simulink model "V2G_System_iPI_Control_Optimized"  (R2025a)
settings: Solver=VariableStepAuto  StartTime=0.0  StopTime=1  RelTol=1e-3
undefined symbols (not defined in the file or in its folder): alpha, Ion, Ki, Kp, Lithium
libraries: spsSeriesRLCBranchLib x16, spsIGBTDiodeLib x12, spsCurrentMeasurementLib x6, slpidlib x4, spsBatteryLib x3, spsPWMGeneratorDCDCLib x3, spsAlphaBetaZerotodq0Lib x3, spsPWMGenerator2LevelLib x1, spsabctoAlphaBetaZeroLib x1, spsdq0toabcLib x1, simulink x1, spsThreePhaseVIMeasurementLib x1
settings Model: Creator=volet  LastModifiedBy=Nripace

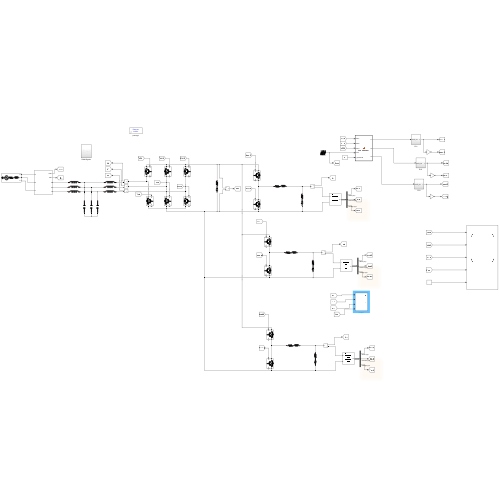
[thumbnail: Simulink's stored preview of the top-level diagram]
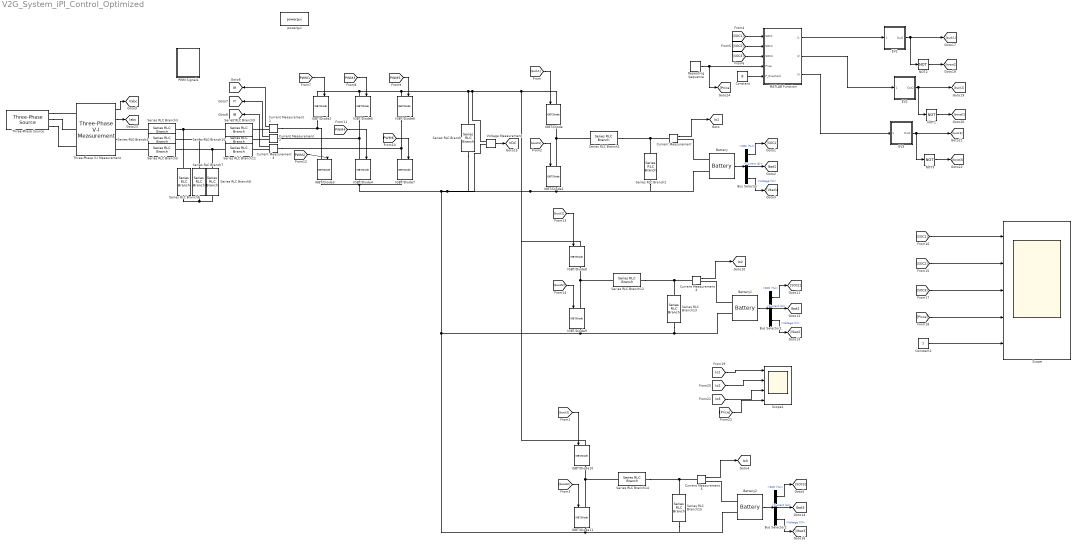
== system V2G_System_iPI_Control_Optimized ==
  Battery : spsBatteryLib/Battery  BatType=Lithium-Ion  NomV=360  NomQ=300  SOC=35  Batt_Tr=1  PresetModel=on  MaxQ=300  MinV=270  FullV=419.0354  Dis_rate=130.4348  R=0.012  Normal_OP=271.3043  expZone="[388.9389      14.73913]"
  Battery1 : spsBatteryLib/Battery  BatType=Lithium-Ion  NomV=360  NomQ=300  SOC=50  Batt_Tr=1  PresetModel=on  MaxQ=300  MinV=270  FullV=419.0354  Dis_rate=130.4348  R=0.012  Normal_OP=271.3043  expZone="[388.9389      14.73913]"
  Battery2 : spsBatteryLib/Battery  BatType=Lithium-Ion  NomV=360  NomQ=300  SOC=75  Batt_Tr=1  PresetModel=on  MaxQ=300  MinV=270  FullV=419.0354  Dis_rate=130.4348  R=0.012  Normal_OP=271.3043  expZone="[388.9389      14.73913]"
  Bus Selector : BusSelector  OutputSignals=SOC (%),Current (A),Voltage (V)
  Bus Selector1 : BusSelector  OutputSignals=SOC (%),Current (A),Voltage (V)
  Bus Selector2 : BusSelector  OutputSignals=SOC (%),Current (A),Voltage (V)
  Constant : Constant  Value=8
  Constant1 : Constant  Value=7
  Current Measurement{,1..5} (6 alike) : spsCurrentMeasurementLib/Current Measurement  PhasorSimulation=off  OutputType=Complex  PSBequivalent=0
  EV1 : Subsystem
  EV2 : Subsystem
  EV3 : Subsystem
  IGBT/Diode{,1..11} (12 alike) : spsIGBTDiodeLib/IGBT//Diode  Ron=1e-3  Rs=1e5  Cs=inf  Measurements=on
  MATLAB Function : MATLAB Function  TreatAsAtomicUnit=on
  NOT1 : Logic  Operator=NOT  IconShape=distinctive  AllPortsSameDT=off  OutDataTypeStr=boolean
  NOT2 : Logic  Operator=NOT  IconShape=distinctive  AllPortsSameDT=off  OutDataTypeStr=boolean
  NOT3 : Logic  Operator=NOT  IconShape=distinctive  AllPortsSameDT=off  OutDataTypeStr=boolean
  PWM Signals : Subsystem
  Repeating Sequence : simulink/Sources/Repeating Sequence  rep_seq_t=[0 0.1 0.2 0.3 0.4 0.5 0.6 0.7 0.8 0.9 1]  rep_seq_y=[6 3.5 8 4.3 6.7 9 8.4 8.8 11 10 9]
  Scope : Scope  NumInputPorts=5
      settings: ActiveDisplayYMinimum=17.794745633890674  ActiveDisplayYMaximum=17.796976065870169
  Scope1 : Scope  NumInputPorts=4
      settings: ActiveDisplayYMinimum=-282.20581600394803  ActiveDisplayYMaximum=129.45342106737178
  Series RLC Branch : spsSeriesRLCBranchLib/Series RLC Branch  LConnTagsString=__new0  RConnTagsString=__new0  BranchType=RC  Resistance=1e-3  Inductance=1e-3  SetiL0=off  InitialCurrent=0  Capacitance=5600e-6  Setx0=on  InitialVoltage=800  Measurements=None
  Series RLC Branch1 : spsSeriesRLCBranchLib/Series RLC Branch  LConnTagsString=__new0  RConnTagsString=__new0  BranchType=RL  Resistance=1e-4  Inductance=20e-3  SetiL0=off  InitialCurrent=0  Capacitance=1000e-6  Setx0=off  InitialVoltage=0  Measurements=None
  Series RLC Branch{3..5,9..11} (6 alike) : spsSeriesRLCBranchLib/Series RLC Branch  LConnTagsString=__new0  RConnTagsString=__new0  BranchType=L  Resistance=1  Inductance=5e-3  SetiL0=off  InitialCurrent=0  Capacitance=1e-6  Setx0=off  InitialVoltage=0  Measurements=None
  Series RLC Branch12 : spsSeriesRLCBranchLib/Series RLC Branch  LConnTagsString=__new0  RConnTagsString=__new0  BranchType=RL  Resistance=1e-4  Inductance=20e-3  SetiL0=off  InitialCurrent=0  Capacitance=1000e-6  Setx0=off  InitialVoltage=0  Measurements=None
  Series RLC Branch13 : spsSeriesRLCBranchLib/Series RLC Branch  LConnTagsString=__new0  RConnTagsString=__new0  BranchType=RC  Resistance=1e-4  Inductance=1e-3  SetiL0=off  InitialCurrent=0  Capacitance=0.625e-6  Setx0=off  InitialVoltage=0  Measurements=None
  Series RLC Branch14 : spsSeriesRLCBranchLib/Series RLC Branch  LConnTagsString=__new0  RConnTagsString=__new0  BranchType=RL  Resistance=1e-4  Inductance=20e-3  SetiL0=off  InitialCurrent=0  Capacitance=1000e-6  Setx0=off  InitialVoltage=0  Measurements=None
  Series RLC Branch15 : spsSeriesRLCBranchLib/Series RLC Branch  LConnTagsString=__new0  RConnTagsString=__new0  BranchType=RC  Resistance=1e-4  Inductance=1e-3  SetiL0=off  InitialCurrent=0  Capacitance=0.625e-6  Setx0=off  InitialVoltage=0  Measurements=None
  Series RLC Branch2 : spsSeriesRLCBranchLib/Series RLC Branch  LConnTagsString=__new0  RConnTagsString=__new0  BranchType=RC  Resistance=1e-4  Inductance=1e-3  SetiL0=off  InitialCurrent=0  Capacitance=0.625e-6  Setx0=off  InitialVoltage=0  Measurements=None
  Series RLC Branch6 : spsSeriesRLCBranchLib/Series RLC Branch  LConnTagsString=__new0  RConnTagsString=__new0  BranchType=C  Resistance=1  Inductance=5e-3  SetiL0=off  InitialCurrent=0  Capacitance=30e-6  Setx0=off  InitialVoltage=0  Measurements=None
  Series RLC Branch7 : spsSeriesRLCBranchLib/Series RLC Branch  LConnTagsString=__new0  RConnTagsString=__new0  BranchType=C  Resistance=1  Inductance=5e-3  SetiL0=off  InitialCurrent=0  Capacitance=30e-6  Setx0=off  InitialVoltage=0  Measurements=None
  Series RLC Branch8 : spsSeriesRLCBranchLib/Series RLC Branch  LConnTagsString=__new0  RConnTagsString=__new0  BranchType=C  Resistance=1  Inductance=5e-3  SetiL0=off  InitialCurrent=0  Capacitance=30e-6  Setx0=off  InitialVoltage=0  Measurements=None
  Three-Phase V-I Measurement : spsThreePhaseVIMeasurementLib/Three-Phase V-I Measurement  VoltageMeasurement=phase-to-ground  SetLabelV=off  LabelV=Vabc  Vpu=off  VpuLL=off  CurrentMeasurement=yes  SetLabelI=off  LabelI=Iabc  Ipu=off  Pbase=100e6  Vbase=500e3  OutputType=Complex  PhasorSimulation=off  PSBequivalent=0
  Three-Phase Source : spsThreePhaseSourceLib/Three-Phase Source  InternalConnection=Yg  VoltagePhases=off  Voltage=415  PhaseAngle=0  Voltage_phases=[25e3 25e3 25e3]/sqrt(3)  PhaseAngles_phases=[0 -120 +120]  Frequency=50  NonIdealSource=on  SpecifyImpedance=off  Resistance=0.8929e-3  Inductance=16.58e-9  ShortCircuitLevel=100e6  BaseVoltage=415  XRratio=7  BusType=swing  Pref=10e3  Qref=0  Prefabc=[10e3, 10e3, 10e3]  Qrefabc=[0, 0, 0]  Qmin=-inf  Qmax=inf
  Voltage Measurement : spsVoltageMeasurementLib/Voltage Measurement  PhasorSimulation=off  OutputType=Complex  PSBequivalent=0
  powergui : sps_lib/powergui  Priority=1  SimulationMode=Discrete  SampleTime=1e-6  frequency=60  Iterations=50  frequencyindice=0  Pbase=100e6  ErrMax=1e-4  UnitsV=kV  UnitsW=MW  buscounter=0  FunctionMessages=off  echomessages=off  EnableUseOfTLC=off  CurrentSourceSwitches=off  DisableSnubberDevices=off  DisableRonSwitches=off  DisableVfSwitches=off  DisplayEquations=off  AutomaticDiscreteSolvers=off  SolverType=Tustin/Backward Euler (TBE)  Interpol=off  ExternalGateDelay=off  methode=off  Ts=100  x0status=blocks  SPID=on  SwTol=0  HookPort=off  NonlinearTolerance=1e-4  nMaxIteration=100  ContinueOnMaxIteration=off  RestoreLinks=warning  ResistiveCurrentMeasurement=off  Frange=[0:2:500]  Ylog=off  Xlog=on  ShowGrid=off  save=off  variable=ZData  structure=0  ZoomFFT=off  StartTime=0.0  cycles=1  DisplayStyle=1  fundamental=60  FreqAxis=off  MaxFrequency=1000  frequencyindicesteady=1  RmsSteady=1  display=off
  tag scope: IB=global, IR=global, IY=global, Iabc=global, Ibat1=global, Ibat2=global, Ibat3=global, Io1=global, Io2=global, Io3=global, VDC=global, Vabc=global
  wires:
  [boost3] -> IGBT/Diode11/1
  [Io3] -> Scope1/3
  Voltage Measurement/1 -> [VDC]
  [PWM3] -> IGBT/Diode5/1
  Bus Selector2/1 -> [SOC3]  "<SOC (%)>"
  Bus Selector2/3 -> [Vbat3]  "<Voltage (V)>"
  [PWM5] -> IGBT/Diode6/1
  [PWM4] -> IGBT/Diode4/1
  [SOC3] -> Scope/3
  MATLAB Function/3(I3) -> EV3/1(Price_ref)
  Three-Phase V-I Measurement/1 -> [Vabc]
  Bus Selector2/2 -> [Ibat3]  "<Current (A)>"
  Current Measurement1/1 -> [IR]
  [Io1] -> Scope1/1
  Bus Selector1/3 -> [Vbat2]  "<Voltage (V)>"
  [SOC3] -> MATLAB Function/3(SOC3)
  Current Measurement4/1 -> [Io2]
  Bus Selector/3 -> [Vbat1]  "<Voltage (V)>"
  EV1/1(Out2) -> [buck1], NOT2/1
  [boost2] -> IGBT/Diode9/1
  MATLAB Function/2(I2) -> EV2/1(Price_ref)
  NOT1/1 -> [boost2]
  [SOC2] -> Scope/2
  [boost1] -> IGBT/Diode1/1
  EV3/1(Out2) -> [buck3], NOT3/1
  Bus Selector/2 -> [Ibat1]  "<Current (A)>"
  [PWM6] -> IGBT/Diode7/1
  Repeating Sequence/1 -> MATLAB Function/4(Price), [Price]
  Three-Phase V-I Measurement/2 -> [Iabc]
  [SOC1] -> MATLAB Function/1(SOC1)
  Constant/1 -> MATLAB Function/5(P_threshold)
  NOT3/1 -> [boost3]
  Bus Selector/1 -> [SOC1]  "<SOC (%)>"
  NOT2/1 -> [boost1]
  [buck2] -> IGBT/Diode8/1
  [Price] -> Scope/4
  Bus Selector1/1 -> [SOC2]  "<SOC (%)>"
  [SOC1] -> Scope/1
  Current Measurement3/1 -> [IB]
  [buck3] -> IGBT/Diode10/1
  MATLAB Function/1(I1) -> EV1/1(Price_ref)
  Current Measurement2/1 -> [IY]
  Battery2/1 -> Bus Selector2/1
  Current Measurement/1 -> [Io1]
  [PWM2] -> IGBT/Diode3/1
  Battery/1 -> Bus Selector/1
  Current Measurement5/1 -> [Io3]
  [Io2] -> Scope1/2
  Bus Selector1/2 -> [Ibat2]  "<Current (A)>"
  [SOC2] -> MATLAB Function/2(SOC2)
  [PWM1] -> IGBT/Diode2/1
  EV2/1(Out2) -> [buck2], NOT1/1
  Battery1/1 -> Bus Selector1/1
  [buck1] -> IGBT/Diode/1
  Constant1/1 -> Scope/5
  [Price] -> Scope1/4
  connections:
  Series RLC Branch14/RConn1 -- Current Measurement5/LConn1 -- Series RLC Branch15/LConn1
  Series RLC Branch13/RConn1 -- Battery1/LConn2 -- IGBT/Diode9/RConn1 -- IGBT/Diode11/RConn1 -- Battery2/LConn2 -- Series RLC Branch15/RConn1 -- IGBT/Diode3/RConn1 -- IGBT/Diode4/RConn1 -- IGBT/Diode7/RConn1 -- Series RLC Branch/RConn1 -- Voltage Measurement/LConn2 -- Battery/LConn2 -- Series RLC Branch2/RConn1 -- IGBT/Diode1/RConn1
  IGBT/Diode5/LConn1 -- IGBT/Diode10/LConn1 -- IGBT/Diode8/LConn1 -- IGBT/Diode/LConn1 -- Voltage Measurement/LConn1 -- Series RLC Branch/LConn1 -- IGBT/Diode6/LConn1 -- IGBT/Diode2/LConn1
  IGBT/Diode9/LConn1 -- Series RLC Branch12/LConn1 -- IGBT/Diode8/RConn1
  IGBT/Diode11/LConn1 -- Series RLC Branch14/LConn1 -- IGBT/Diode10/RConn1
  Series RLC Branch6/RConn1 -- Series RLC Branch7/RConn1 -- Series RLC Branch8/RConn1
  IGBT/Diode1/LConn1 -- Series RLC Branch1/LConn1 -- IGBT/Diode/RConn1
  IGBT/Diode5/RConn1 -- Current Measurement2/LConn1 -- IGBT/Diode4/LConn1
  Series RLC Branch3/RConn1 -- Series RLC Branch6/LConn1 -- Series RLC Branch9/LConn1
  IGBT/Diode2/RConn1 -- Current Measurement1/LConn1 -- IGBT/Diode3/LConn1
  Series RLC Branch7/LConn1 -- Series RLC Branch4/RConn1 -- Series RLC Branch10/LConn1
  IGBT/Diode6/RConn1 -- Current Measurement3/LConn1 -- IGBT/Diode7/LConn1
  Series RLC Branch8/LConn1 -- Series RLC Branch5/RConn1 -- Series RLC Branch11/LConn1
  Series RLC Branch1/RConn1 -- Current Measurement/LConn1 -- Series RLC Branch2/LConn1
  Series RLC Branch12/RConn1 -- Current Measurement4/LConn1 -- Series RLC Branch13/LConn1
  Current Measurement3/RConn1 -- Series RLC Branch11/RConn1
  Battery/LConn1 -- Current Measurement/RConn1
  Three-Phase Source/RConn3 -- Three-Phase V-I Measurement/LConn3
  Current Measurement2/RConn1 -- Series RLC Branch10/RConn1
  Three-Phase Source/RConn2 -- Three-Phase V-I Measurement/LConn2
  Series RLC Branch3/LConn1 -- Three-Phase V-I Measurement/RConn1
  Series RLC Branch4/LConn1 -- Three-Phase V-I Measurement/RConn2
  Three-Phase Source/RConn1 -- Three-Phase V-I Measurement/LConn1
  Battery2/LConn1 -- Current Measurement5/RConn1
  Current Measurement1/RConn1 -- Series RLC Branch9/RConn1
  Battery1/LConn1 -- Current Measurement4/RConn1
  Series RLC Branch5/LConn1 -- Three-Phase V-I Measurement/RConn3

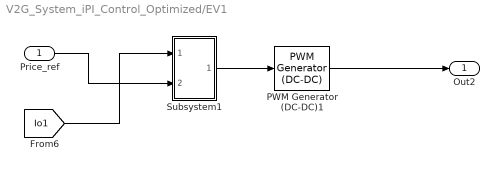
== system V2G_System_iPI_Control_Optimized/EV1 ==
  Price_ref : Inport
  PWM Generator (DC-DC)1 : spsPWMGeneratorDCDCLib/PWM Generator (DC-DC)  Fsw=10000  Ts=0
  Subsystem1 : Subsystem
  Out2 : Outport  VectorParamsAs1DForOutWhenUnconnected=off
  wires:
  Subsystem1/1(Out1) -> PWM Generator (DC-DC)1/1
  PWM Generator (DC-DC)1/1 -> Out2/1
  [Io1] -> Subsystem1/1(Price_ref)
  Price_ref/1 -> Subsystem1/2(In2)

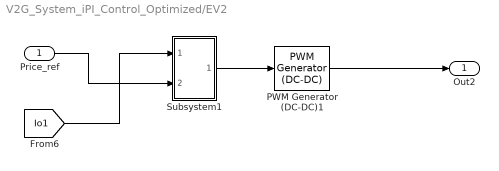
== system V2G_System_iPI_Control_Optimized/EV2 ==
  Price_ref : Inport
  PWM Generator (DC-DC)1 : spsPWMGeneratorDCDCLib/PWM Generator (DC-DC)  Fsw=10000  Ts=0
  Subsystem1 : Subsystem
  Out2 : Outport  VectorParamsAs1DForOutWhenUnconnected=off
  wires:
  Subsystem1/1(Out1) -> PWM Generator (DC-DC)1/1
  PWM Generator (DC-DC)1/1 -> Out2/1
  [Io1] -> Subsystem1/1(Price_ref)
  Price_ref/1 -> Subsystem1/2(In2)

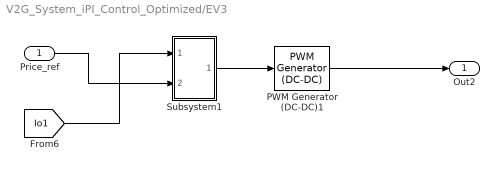
== system V2G_System_iPI_Control_Optimized/EV3 ==
  Price_ref : Inport
  PWM Generator (DC-DC)1 : spsPWMGeneratorDCDCLib/PWM Generator (DC-DC)  Fsw=10000  Ts=0
  Subsystem1 : Subsystem
  Out2 : Outport  VectorParamsAs1DForOutWhenUnconnected=off
  wires:
  Price_ref/1 -> Subsystem1/2(In2)
  [Io1] -> Subsystem1/1(Price_ref)
  PWM Generator (DC-DC)1/1 -> Out2/1
  Subsystem1/1(Out1) -> PWM Generator (DC-DC)1/1

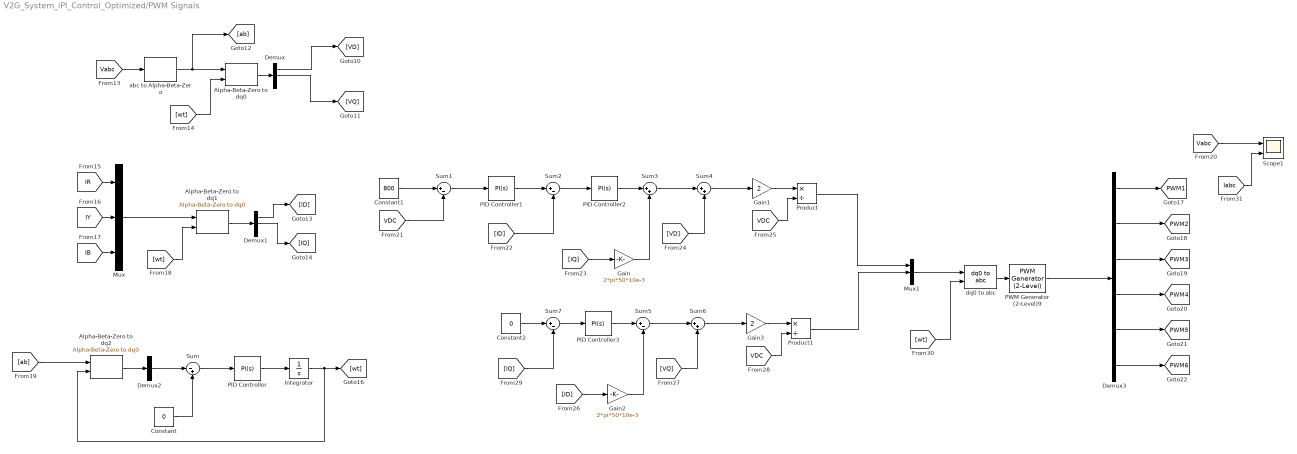
== system V2G_System_iPI_Control_Optimized/PWM Signals ==
  Alpha-Beta-Zero to dq0 : spsAlphaBetaZerotodq0Lib/Alpha-Beta-Zero to dq0  Alignment=90 degrees behind phase A axis
  Alpha-Beta-Zero to dq1 : spsAlphaBetaZerotodq0Lib/Alpha-Beta-Zero to dq0  Alignment=90 degrees behind phase A axis
  Alpha-Beta-Zero to dq2 : spsAlphaBetaZerotodq0Lib/Alpha-Beta-Zero to dq0  Alignment=90 degrees behind phase A axis
  Constant : Constant  Value=0
  Constant1 : Constant  Value=800
  Constant2 : Constant  Value=0
  Demux : Demux  Outputs=3
  Demux1 : Demux  Outputs=3
  Demux2 : Demux  Outputs=3
  Demux3 : Demux  Outputs=6
  Gain : Gain  Gain=2*pi*50*10e-3
  Gain1 : Gain  Gain=2
  Gain2 : Gain  Gain=2*pi*50*10e-3
  Gain3 : Gain  Gain=2
  Integrator : Integrator
  Mux : Mux  Inputs=3
  Mux1 : Mux  Inputs=3
  PID Controller : slpidlib/PID Controller  Controller=PI  Form=Parallel  TimeDomain=Continuous-time  UseExternalTs=off  SampleTime=-1  IntegratorMethod=Forward Euler  FilterMethod=Forward Euler  ControllerParametersSource=internal  P=10  I=50000  UseKiTs=off  D=0  UseExternalDerivativeSource=off  N=100  UseFilter=on  TunerSelectOption=Transfer Function Based (PID Tuner App)  InitialConditionSource=internal  InitialConditionForIntegrator=0  InitialConditionForFilter=0  DifferentiatorICPrevScaledInput=0  ExternalReset=none  TrackingMode=off  Kt=1  LimitOutput=off  SatLimitsSource=internal  UpperSaturationLimit=inf  LowerSaturationLimit=-inf  LinearizeAsGain=on  AntiWindupMode=none  Kb=1  LimitIntegrator=off  UpperIntegratorSaturationLimit=inf  LowerIntegratorSaturationLimit=-inf  POutMin=[]  POutMax=[]  IOutMin=[]  IOutMax=[]  DOutMin=[]  DOutMax=[]  NOutMin=[]  NOutMax=[]  SumOutMin=[]  SumOutMax=[]  SaturationOutMin=[]  SaturationOutMax=[]  PParamMin=[]  PParamMax=[]  IParamMin=[]  IParamMax=[]  DParamMin=[]  DParamMax=[]  NParamMin=[]  NParamMax=[]  KbParamMin=[]  KbParamMax=[]  KtParamMin=[]  KtParamMax=[]  KbOutMin=[]  KbOutMax=[]  KtOutMin=[]  KtOutMax=[]  IntegratorOutMin=[]  IntegratorOutMax=[]  FilterOutMin=[]  FilterOutMax=[]  SumI1OutMin=[]  SumI1OutMax=[]  SumI2OutMin=[]  SumI2OutMax=[]  SumI3OutMin=[]  SumI3OutMax=[]  SumI4OutMin=[]  SumI4OutMax=[]  SumDOutMin=[]  SumDOutMax=[]  DifferentiatorOutMin=[]  DifferentiatorOutMax=[]  FilterDiffOutCoefMin=[]  FilterDiffOutCoefMax=[]  ReciprocalOutMin=[]  ReciprocalOutMax=[]  SumDenOutMin=[]  SumDenOutMax=[]  SumNumOutMin=[]  SumNumOutMax=[]  DivideOutMin=[]  DivideOutMax=[]  UdiffTsProdOutMin=[]  UdiffTsProdOutMax=[]  NTsProdOutMin=[]  NTsProdOutMax=[]  UintegralTsProdOutMin=[]  UintegralTsProdOutMax=[]  UngainTsProdOutMin=[]  UngainTsProdOutMax=[]  ClampingZeroOutDataTypeStr=Inherit: Inherit via back propagation  ClampingZeroOutMin=[]  ClampingZeroOutMax=[]  FilterDenConstantOutDataTypeStr=Inherit: Inherit via back propagation  FilterDenConstantOutMin=[]  FilterDenConstantOutMax=[]  PCopyOutDataTypeStr=Inherit: Inherit via back propagation  PCopyOutMin=[]  PCopyOutMax=[]  NCopyOutDataTypeStr=Inherit: Inherit via back propagation  NCopyOutMin=[]  NCopyOutMax=[]  IntegratorContinuousStateAttributes=''  IntegratorStateMustResolveToSignalObject=off  IntegratorRTWStateStorageClass=Auto  FilterContinuousStateAttributes=''  FilterStateMustResolveToSignalObject=off  FilterRTWStateStorageClass=Auto  ParallelPVariant=InternalParameters  IdealPVariant=Disabled  IVariant=InternalParameters  DVariant=Disabled  IntegratorVariant=Continuous  SatVariant=Disabled  AWVariant=Passthrough  PCopyVariant=Disabled  TRVariant=Disabled  FdbkBlocksVariant=Forward  IdealPFdbkVariant=Disabled  SatFdbkVariant=Disabled  DerivativeFilterVariant=Disabled  NVariant=Disabled  NCopyVariant=Disabled_SignalSpec  FilterICVariant=Disabled  IntegratorICVariant=InternalICs  ExternalResetVariant=Disabled  TRSumVariant=Passthrough  SumFdbkVariant=Disabled  SumVariant=Sum_PI  TsampFilterVariant=InternalTs  TsampNgainVariant=Passthrough  TsampIntegralVariant=Disabled_SignalSpec  ExternalSaturationOutDataTypeStr=Inherit: Same as second input  DerivativeSourceVariant=Disabled  PreIntVariant=InternalPreInt
  PID Controller1 : slpidlib/PID Controller  Controller=PI  Form=Parallel  TimeDomain=Continuous-time  UseExternalTs=off  SampleTime=-1  IntegratorMethod=Forward Euler  FilterMethod=Forward Euler  ControllerParametersSource=internal  P=0.5  I=5  UseKiTs=off  D=0  UseExternalDerivativeSource=off  N=100  UseFilter=on  TunerSelectOption=Transfer Function Based (PID Tuner App)  InitialConditionSource=internal  InitialConditionForIntegrator=0  InitialConditionForFilter=0  DifferentiatorICPrevScaledInput=0  ExternalReset=none  TrackingMode=off  Kt=1  LimitOutput=off  SatLimitsSource=internal  UpperSaturationLimit=inf  LowerSaturationLimit=-inf  LinearizeAsGain=on  AntiWindupMode=none  Kb=1  LimitIntegrator=off  UpperIntegratorSaturationLimit=inf  LowerIntegratorSaturationLimit=-inf  POutMin=[]  POutMax=[]  IOutMin=[]  IOutMax=[]  DOutMin=[]  DOutMax=[]  NOutMin=[]  NOutMax=[]  SumOutMin=[]  SumOutMax=[]  SaturationOutMin=[]  SaturationOutMax=[]  PParamMin=[]  PParamMax=[]  IParamMin=[]  IParamMax=[]  DParamMin=[]  DParamMax=[]  NParamMin=[]  NParamMax=[]  KbParamMin=[]  KbParamMax=[]  KtParamMin=[]  KtParamMax=[]  KbOutMin=[]  KbOutMax=[]  KtOutMin=[]  KtOutMax=[]  IntegratorOutMin=[]  IntegratorOutMax=[]  FilterOutMin=[]  FilterOutMax=[]  SumI1OutMin=[]  SumI1OutMax=[]  SumI2OutMin=[]  SumI2OutMax=[]  SumI3OutMin=[]  SumI3OutMax=[]  SumI4OutMin=[]  SumI4OutMax=[]  SumDOutMin=[]  SumDOutMax=[]  DifferentiatorOutMin=[]  DifferentiatorOutMax=[]  FilterDiffOutCoefMin=[]  FilterDiffOutCoefMax=[]  ReciprocalOutMin=[]  ReciprocalOutMax=[]  SumDenOutMin=[]  SumDenOutMax=[]  SumNumOutMin=[]  SumNumOutMax=[]  DivideOutMin=[]  DivideOutMax=[]  UdiffTsProdOutMin=[]  UdiffTsProdOutMax=[]  NTsProdOutMin=[]  NTsProdOutMax=[]  UintegralTsProdOutMin=[]  UintegralTsProdOutMax=[]  UngainTsProdOutMin=[]  UngainTsProdOutMax=[]  ClampingZeroOutDataTypeStr=Inherit: Inherit via back propagation  ClampingZeroOutMin=[]  ClampingZeroOutMax=[]  FilterDenConstantOutDataTypeStr=Inherit: Inherit via back propagation  FilterDenConstantOutMin=[]  FilterDenConstantOutMax=[]  PCopyOutDataTypeStr=Inherit: Inherit via back propagation  PCopyOutMin=[]  PCopyOutMax=[]  NCopyOutDataTypeStr=Inherit: Inherit via back propagation  NCopyOutMin=[]  NCopyOutMax=[]  IntegratorContinuousStateAttributes=''  IntegratorStateMustResolveToSignalObject=off  IntegratorRTWStateStorageClass=Auto  FilterContinuousStateAttributes=''  FilterStateMustResolveToSignalObject=off  FilterRTWStateStorageClass=Auto  ParallelPVariant=InternalParameters  IdealPVariant=Disabled  IVariant=InternalParameters  DVariant=Disabled  IntegratorVariant=Continuous  SatVariant=Disabled  AWVariant=Passthrough  PCopyVariant=Disabled  TRVariant=Disabled  FdbkBlocksVariant=Forward  IdealPFdbkVariant=Disabled  SatFdbkVariant=Disabled  DerivativeFilterVariant=Disabled  NVariant=Disabled  NCopyVariant=Disabled_SignalSpec  FilterICVariant=Disabled  IntegratorICVariant=InternalICs  ExternalResetVariant=Disabled  TRSumVariant=Passthrough  SumFdbkVariant=Disabled  SumVariant=Sum_PI  TsampFilterVariant=InternalTs  TsampNgainVariant=Passthrough  TsampIntegralVariant=Disabled_SignalSpec  ExternalSaturationOutDataTypeStr=Inherit: Same as second input  DerivativeSourceVariant=Disabled  PreIntVariant=InternalPreInt
  PID Controller2 : slpidlib/PID Controller  Controller=PI  Form=Parallel  TimeDomain=Continuous-time  UseExternalTs=off  SampleTime=-1  IntegratorMethod=Forward Euler  FilterMethod=Forward Euler  ControllerParametersSource=internal  P=25  I=500  UseKiTs=off  D=0  UseExternalDerivativeSource=off  N=100  UseFilter=on  TunerSelectOption=Transfer Function Based (PID Tuner App)  InitialConditionSource=internal  InitialConditionForIntegrator=0  InitialConditionForFilter=0  DifferentiatorICPrevScaledInput=0  ExternalReset=none  TrackingMode=off  Kt=1  LimitOutput=off  SatLimitsSource=internal  UpperSaturationLimit=inf  LowerSaturationLimit=-inf  LinearizeAsGain=on  AntiWindupMode=none  Kb=1  LimitIntegrator=off  UpperIntegratorSaturationLimit=inf  LowerIntegratorSaturationLimit=-inf  POutMin=[]  POutMax=[]  IOutMin=[]  IOutMax=[]  DOutMin=[]  DOutMax=[]  NOutMin=[]  NOutMax=[]  SumOutMin=[]  SumOutMax=[]  SaturationOutMin=[]  SaturationOutMax=[]  PParamMin=[]  PParamMax=[]  IParamMin=[]  IParamMax=[]  DParamMin=[]  DParamMax=[]  NParamMin=[]  NParamMax=[]  KbParamMin=[]  KbParamMax=[]  KtParamMin=[]  KtParamMax=[]  KbOutMin=[]  KbOutMax=[]  KtOutMin=[]  KtOutMax=[]  IntegratorOutMin=[]  IntegratorOutMax=[]  FilterOutMin=[]  FilterOutMax=[]  SumI1OutMin=[]  SumI1OutMax=[]  SumI2OutMin=[]  SumI2OutMax=[]  SumI3OutMin=[]  SumI3OutMax=[]  SumI4OutMin=[]  SumI4OutMax=[]  SumDOutMin=[]  SumDOutMax=[]  DifferentiatorOutMin=[]  DifferentiatorOutMax=[]  FilterDiffOutCoefMin=[]  FilterDiffOutCoefMax=[]  ReciprocalOutMin=[]  ReciprocalOutMax=[]  SumDenOutMin=[]  SumDenOutMax=[]  SumNumOutMin=[]  SumNumOutMax=[]  DivideOutMin=[]  DivideOutMax=[]  UdiffTsProdOutMin=[]  UdiffTsProdOutMax=[]  NTsProdOutMin=[]  NTsProdOutMax=[]  UintegralTsProdOutMin=[]  UintegralTsProdOutMax=[]  UngainTsProdOutMin=[]  UngainTsProdOutMax=[]  ClampingZeroOutDataTypeStr=Inherit: Inherit via back propagation  ClampingZeroOutMin=[]  ClampingZeroOutMax=[]  FilterDenConstantOutDataTypeStr=Inherit: Inherit via back propagation  FilterDenConstantOutMin=[]  FilterDenConstantOutMax=[]  PCopyOutDataTypeStr=Inherit: Inherit via back propagation  PCopyOutMin=[]  PCopyOutMax=[]  NCopyOutDataTypeStr=Inherit: Inherit via back propagation  NCopyOutMin=[]  NCopyOutMax=[]  IntegratorContinuousStateAttributes=''  IntegratorStateMustResolveToSignalObject=off  IntegratorRTWStateStorageClass=Auto  FilterContinuousStateAttributes=''  FilterStateMustResolveToSignalObject=off  FilterRTWStateStorageClass=Auto  ParallelPVariant=InternalParameters  IdealPVariant=Disabled  IVariant=InternalParameters  DVariant=Disabled  IntegratorVariant=Continuous  SatVariant=Disabled  AWVariant=Passthrough  PCopyVariant=Disabled  TRVariant=Disabled  FdbkBlocksVariant=Forward  IdealPFdbkVariant=Disabled  SatFdbkVariant=Disabled  DerivativeFilterVariant=Disabled  NVariant=Disabled  NCopyVariant=Disabled_SignalSpec  FilterICVariant=Disabled  IntegratorICVariant=InternalICs  ExternalResetVariant=Disabled  TRSumVariant=Passthrough  SumFdbkVariant=Disabled  SumVariant=Sum_PI  TsampFilterVariant=InternalTs  TsampNgainVariant=Passthrough  TsampIntegralVariant=Disabled_SignalSpec  ExternalSaturationOutDataTypeStr=Inherit: Same as second input  DerivativeSourceVariant=Disabled  PreIntVariant=InternalPreInt
  PID Controller3 : slpidlib/PID Controller  Controller=PI  Form=Parallel  TimeDomain=Continuous-time  UseExternalTs=off  SampleTime=-1  IntegratorMethod=Forward Euler  FilterMethod=Forward Euler  ControllerParametersSource=internal  P=25  I=500  UseKiTs=off  D=0  UseExternalDerivativeSource=off  N=100  UseFilter=on  TunerSelectOption=Transfer Function Based (PID Tuner App)  InitialConditionSource=internal  InitialConditionForIntegrator=0  InitialConditionForFilter=0  DifferentiatorICPrevScaledInput=0  ExternalReset=none  TrackingMode=off  Kt=1  LimitOutput=off  SatLimitsSource=internal  UpperSaturationLimit=inf  LowerSaturationLimit=-inf  LinearizeAsGain=on  AntiWindupMode=none  Kb=1  LimitIntegrator=off  UpperIntegratorSaturationLimit=inf  LowerIntegratorSaturationLimit=-inf  POutMin=[]  POutMax=[]  IOutMin=[]  IOutMax=[]  DOutMin=[]  DOutMax=[]  NOutMin=[]  NOutMax=[]  SumOutMin=[]  SumOutMax=[]  SaturationOutMin=[]  SaturationOutMax=[]  PParamMin=[]  PParamMax=[]  IParamMin=[]  IParamMax=[]  DParamMin=[]  DParamMax=[]  NParamMin=[]  NParamMax=[]  KbParamMin=[]  KbParamMax=[]  KtParamMin=[]  KtParamMax=[]  KbOutMin=[]  KbOutMax=[]  KtOutMin=[]  KtOutMax=[]  IntegratorOutMin=[]  IntegratorOutMax=[]  FilterOutMin=[]  FilterOutMax=[]  SumI1OutMin=[]  SumI1OutMax=[]  SumI2OutMin=[]  SumI2OutMax=[]  SumI3OutMin=[]  SumI3OutMax=[]  SumI4OutMin=[]  SumI4OutMax=[]  SumDOutMin=[]  SumDOutMax=[]  DifferentiatorOutMin=[]  DifferentiatorOutMax=[]  FilterDiffOutCoefMin=[]  FilterDiffOutCoefMax=[]  ReciprocalOutMin=[]  ReciprocalOutMax=[]  SumDenOutMin=[]  SumDenOutMax=[]  SumNumOutMin=[]  SumNumOutMax=[]  DivideOutMin=[]  DivideOutMax=[]  UdiffTsProdOutMin=[]  UdiffTsProdOutMax=[]  NTsProdOutMin=[]  NTsProdOutMax=[]  UintegralTsProdOutMin=[]  UintegralTsProdOutMax=[]  UngainTsProdOutMin=[]  UngainTsProdOutMax=[]  ClampingZeroOutDataTypeStr=Inherit: Inherit via back propagation  ClampingZeroOutMin=[]  ClampingZeroOutMax=[]  FilterDenConstantOutDataTypeStr=Inherit: Inherit via back propagation  FilterDenConstantOutMin=[]  FilterDenConstantOutMax=[]  PCopyOutDataTypeStr=Inherit: Inherit via back propagation  PCopyOutMin=[]  PCopyOutMax=[]  NCopyOutDataTypeStr=Inherit: Inherit via back propagation  NCopyOutMin=[]  NCopyOutMax=[]  IntegratorContinuousStateAttributes=''  IntegratorStateMustResolveToSignalObject=off  IntegratorRTWStateStorageClass=Auto  FilterContinuousStateAttributes=''  FilterStateMustResolveToSignalObject=off  FilterRTWStateStorageClass=Auto  ParallelPVariant=InternalParameters  IdealPVariant=Disabled  IVariant=InternalParameters  DVariant=Disabled  IntegratorVariant=Continuous  SatVariant=Disabled  AWVariant=Passthrough  PCopyVariant=Disabled  TRVariant=Disabled  FdbkBlocksVariant=Forward  IdealPFdbkVariant=Disabled  SatFdbkVariant=Disabled  DerivativeFilterVariant=Disabled  NVariant=Disabled  NCopyVariant=Disabled_SignalSpec  FilterICVariant=Disabled  IntegratorICVariant=InternalICs  ExternalResetVariant=Disabled  TRSumVariant=Passthrough  SumFdbkVariant=Disabled  SumVariant=Sum_PI  TsampFilterVariant=InternalTs  TsampNgainVariant=Passthrough  TsampIntegralVariant=Disabled_SignalSpec  ExternalSaturationOutDataTypeStr=Inherit: Same as second input  DerivativeSourceVariant=Disabled  PreIntVariant=InternalPreInt
  PWM Generator (2-Level)9 : spsPWMGenerator2LevelLib/PWM Generator (2-Level)  ModulatorType=Three-phase bridge (6 pulses)  ModulatorMode=Unsynchronized  Fc=10e3  Pc=90  nF=27  MinMax="[ -1  1 ]"  SamplingTechnique=Natural  ModulatingSignals=off  m=0.8  Freq=60  Phase=0  Ts=0  ShowCarrierOutport=off
  Product : Product  Inputs=*/
  Product1 : Product  Inputs=*/
  Scope1 : Scope  NumInputPorts=2
      settings: ActiveDisplayYMinimum=-423.55760137027858  ActiveDisplayYMaximum=423.55760137041966  DataLoggingVariableName=ScopeData2
  Sum : Sum  Inputs=|-+
  Sum{1..2,5,7} (4 alike) : Sum  Inputs=|+-
  Sum3 : Sum  Inputs=|++
  Sum4 : Sum  Inputs=|++
  Sum6 : Sum  Inputs=|++
  abc to Alpha-Beta-Zero : spsabctoAlphaBetaZeroLib/abc to Alpha-Beta-Zero
  dq0 to abc : spsdq0toabcLib/dq0 to abc  Alignment=90 degrees behind phase A axis
  tag scope: PWM1=global, PWM2=global, PWM3=global, PWM4=global, PWM5=global, PWM6=global
  wires:
  [ID] -> Sum2/2
  Gain/1 -> Sum3/2
  Alpha-Beta-Zero to dq0/1 -> Demux/1
  Demux3/1 -> [PWM1]
  Constant1/1 -> Sum1/1
  Demux/2 -> [VQ]
  Sum6/1 -> Gain3/1
  [Vabc] -> abc to Alpha-Beta-Zero/1
  dq0 to abc/1 -> PWM Generator (2-Level)9/1
  [wt] -> dq0 to abc/2
  Demux3/6 -> [PWM6]
  [wt] -> Alpha-Beta-Zero to dq0/2
  PID Controller3/1 -> Sum5/1
  Sum5/1 -> Sum6/1
  abc to Alpha-Beta-Zero/1 -> [ab], Alpha-Beta-Zero to dq0/1
  [IQ] -> Sum7/2
  [IY] -> Mux/2
  Alpha-Beta-Zero to dq2/1 -> Demux2/1
  Sum1/1 -> PID Controller1/1
  [Iabc] -> Scope1/2
  Mux/1 -> Alpha-Beta-Zero to dq1/1
  Mux1/1 -> dq0 to abc/1
  Demux2/2 -> Sum/1
  Product1/1 -> Mux1/2
  Product/1 -> Mux1/1
  Constant/1 -> Sum/2
  Gain2/1 -> Sum5/2
  Demux3/4 -> [PWM4]
  [wt] -> Alpha-Beta-Zero to dq1/2
  PID Controller1/1 -> Sum2/1
  PID Controller/1 -> Integrator/1
  Sum/1 -> PID Controller/1
  [IR] -> Mux/1
  Demux3/5 -> [PWM5]
  Integrator/1 -> Alpha-Beta-Zero to dq2/2, [wt]
  [VDC] -> Sum1/2
  Sum4/1 -> Gain1/1
  Demux1/1 -> [ID]
  [VQ] -> Sum6/2
  [ab] -> Alpha-Beta-Zero to dq2/1
  Gain1/1 -> Product/1
  [VDC] -> Product1/2
  Demux3/2 -> [PWM2]
  [Vabc] -> Scope1/1
  [VDC] -> Product/2
  [IB] -> Mux/3
  Demux1/2 -> [IQ]
  [VD] -> Sum4/2
  Demux/1 -> [VD]
  Demux3/3 -> [PWM3]
  Sum3/1 -> Sum4/1
  PWM Generator (2-Level)9/1 -> Demux3/1
  Gain3/1 -> Product1/1
  Constant2/1 -> Sum7/1
  PID Controller2/1 -> Sum3/1
  Sum2/1 -> PID Controller2/1
  [ID] -> Gain2/1
  Sum7/1 -> PID Controller3/1
  Alpha-Beta-Zero to dq1/1 -> Demux1/1
  [IQ] -> Gain/1

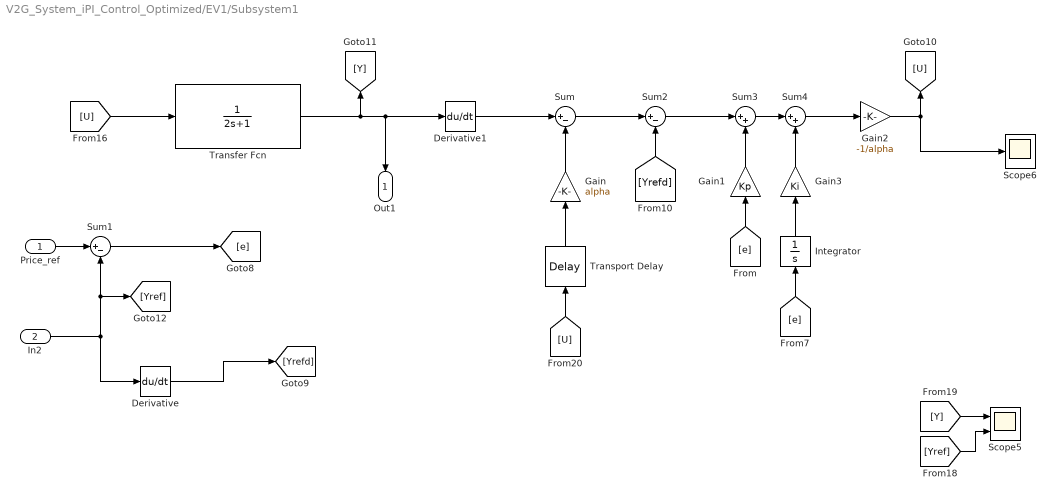
== system V2G_System_iPI_Control_Optimized/EV1/Subsystem1 ==
  Price_ref : Inport
  In2 : Inport  Port=2
  Derivative : Derivative
  Derivative1 : Derivative
  Gain : Gain  Gain=alpha
  Gain1 : Gain  Gain=Kp
  Gain2 : Gain  Gain=-1/alpha
  Gain3 : Gain  Gain=Ki
  Integrator : Integrator
  Scope5 : Scope  NumInputPorts=2
      settings: ActiveDisplayYMinimum=-0.12496149680200519  ActiveDisplayYMaximum=1.1246534712180469  DataLoggingVariableName=ScopeData5
  Scope6 : Scope
      settings: ActiveDisplayYMinimum=-1.1227052321097705E+12  ActiveDisplayYMaximum=9.61894066880864E+12  DataLoggingVariableName=ScopeData6
  Sum : Sum  Inputs=|+-
  Sum1 : Sum  Inputs=|+-
  Sum2 : Sum  Inputs=|+-
  Sum3 : Sum  Inputs=|++
  Sum4 : Sum  Inputs=|++
  Transfer Fcn : TransferFcn  Denominator=[2 1]
  Transport Delay : TransportDelay
  Out1 : Outport  VectorParamsAs1DForOutWhenUnconnected=off
  wires:
  [e] -> Gain1/1
  Sum2/1 -> Sum3/1
  [U] -> Transfer Fcn/1
  Derivative/1 -> [Yrefd]
  Gain2/1 -> [U], Scope6/1
  [U] -> Transport Delay/1
  Gain/1 -> Sum/2
  Transport Delay/1 -> Gain/1
  In2/1 -> [Yref], Sum1/2, Derivative/1
  Transfer Fcn/1 -> [Y], Derivative1/1, Out1/1
  [Yref] -> Scope5/2
  Sum/1 -> Sum2/1
  Sum1/1 -> [e]
  Gain1/1 -> Sum3/2
  Derivative1/1 -> Sum/1
  Price_ref/1 -> Sum1/1
  [Y] -> Scope5/1
  [Yrefd] -> Sum2/2
  [e] -> Integrator/1
  Sum4/1 -> Gain2/1
  Integrator/1 -> Gain3/1
  Sum3/1 -> Sum4/1
  Gain3/1 -> Sum4/2

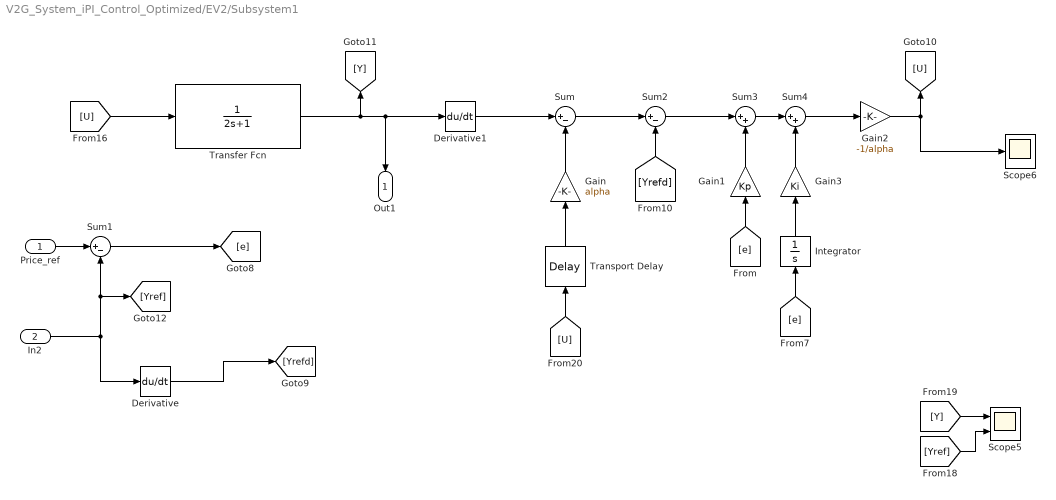
== system V2G_System_iPI_Control_Optimized/EV2/Subsystem1 ==
  Price_ref : Inport
  In2 : Inport  Port=2
  Derivative : Derivative
  Derivative1 : Derivative
  Gain : Gain  Gain=alpha
  Gain1 : Gain  Gain=Kp
  Gain2 : Gain  Gain=-1/alpha
  Gain3 : Gain  Gain=Ki
  Integrator : Integrator
  Scope5 : Scope  NumInputPorts=2
      settings: ActiveDisplayYMinimum=-0.12496149680200519  ActiveDisplayYMaximum=1.1246534712180469  DataLoggingVariableName=ScopeData5
  Scope6 : Scope
      settings: ActiveDisplayYMinimum=-1.1227052321097705E+12  ActiveDisplayYMaximum=9.61894066880864E+12  DataLoggingVariableName=ScopeData6
  Sum : Sum  Inputs=|+-
  Sum1 : Sum  Inputs=|+-
  Sum2 : Sum  Inputs=|+-
  Sum3 : Sum  Inputs=|++
  Sum4 : Sum  Inputs=|++
  Transfer Fcn : TransferFcn  Denominator=[2 1]
  Transport Delay : TransportDelay
  Out1 : Outport  VectorParamsAs1DForOutWhenUnconnected=off
  wires:
  [e] -> Gain1/1
  Sum2/1 -> Sum3/1
  [U] -> Transfer Fcn/1
  Derivative/1 -> [Yrefd]
  Gain2/1 -> [U], Scope6/1
  [U] -> Transport Delay/1
  Gain/1 -> Sum/2
  Transport Delay/1 -> Gain/1
  In2/1 -> [Yref], Sum1/2, Derivative/1
  Transfer Fcn/1 -> [Y], Derivative1/1, Out1/1
  [Yref] -> Scope5/2
  Sum/1 -> Sum2/1
  Sum1/1 -> [e]
  Gain1/1 -> Sum3/2
  Derivative1/1 -> Sum/1
  Price_ref/1 -> Sum1/1
  [Y] -> Scope5/1
  [Yrefd] -> Sum2/2
  [e] -> Integrator/1
  Sum4/1 -> Gain2/1
  Integrator/1 -> Gain3/1
  Sum3/1 -> Sum4/1
  Gain3/1 -> Sum4/2

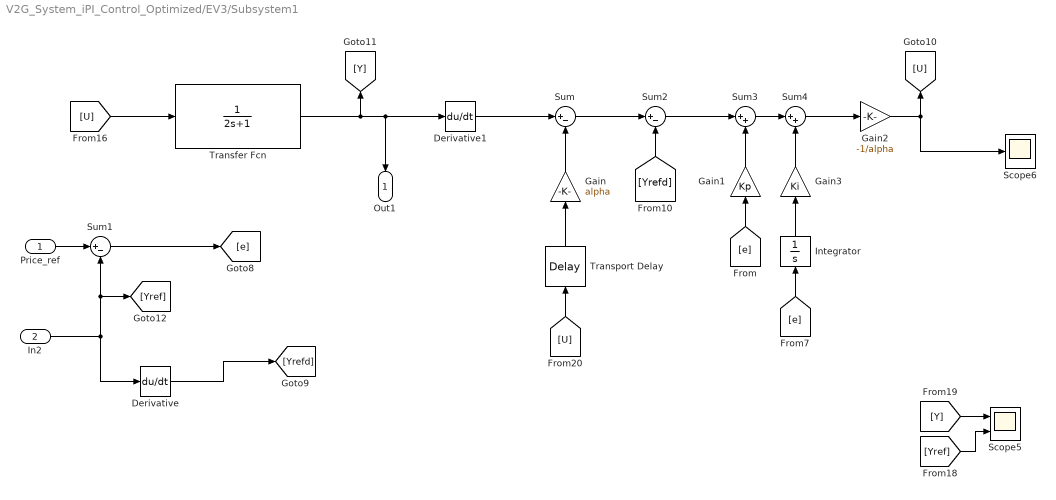
== system V2G_System_iPI_Control_Optimized/EV3/Subsystem1 ==
  Price_ref : Inport
  In2 : Inport  Port=2
  Derivative : Derivative
  Derivative1 : Derivative
  Gain : Gain  Gain=alpha
  Gain1 : Gain  Gain=Kp
  Gain2 : Gain  Gain=-1/alpha
  Gain3 : Gain  Gain=Ki
  Integrator : Integrator
  Scope5 : Scope  NumInputPorts=2
      settings: ActiveDisplayYMinimum=-0.12496149680200519  ActiveDisplayYMaximum=1.1246534712180469  DataLoggingVariableName=ScopeData5
  Scope6 : Scope
      settings: ActiveDisplayYMinimum=-1.1227052321097705E+12  ActiveDisplayYMaximum=9.61894066880864E+12  DataLoggingVariableName=ScopeData6
  Sum : Sum  Inputs=|+-
  Sum1 : Sum  Inputs=|+-
  Sum2 : Sum  Inputs=|+-
  Sum3 : Sum  Inputs=|++
  Sum4 : Sum  Inputs=|++
  Transfer Fcn : TransferFcn  Denominator=[2 1]
  Transport Delay : TransportDelay
  Out1 : Outport  VectorParamsAs1DForOutWhenUnconnected=off
  wires:
  Gain3/1 -> Sum4/2
  Sum3/1 -> Sum4/1
  Integrator/1 -> Gain3/1
  Sum4/1 -> Gain2/1
  [e] -> Integrator/1
  [Yrefd] -> Sum2/2
  [Y] -> Scope5/1
  Price_ref/1 -> Sum1/1
  Derivative1/1 -> Sum/1
  Gain1/1 -> Sum3/2
  Sum1/1 -> [e]
  Sum/1 -> Sum2/1
  [Yref] -> Scope5/2
  Transfer Fcn/1 -> Out1/1, Derivative1/1, [Y]
  In2/1 -> Derivative/1, Sum1/2, [Yref]
  Transport Delay/1 -> Gain/1
  Gain/1 -> Sum/2
  [U] -> Transport Delay/1
  Gain2/1 -> Scope6/1, [U]
  Derivative/1 -> [Yrefd]
  [U] -> Transfer Fcn/1
  Sum2/1 -> Sum3/1
  [e] -> Gain1/1

== matlab function V2G_System_iPI_Control_Optimized/MATLAB Function ==
  data: SOC1 input; I1 output; SOC2 input; SOC3 input; Price input; P_threshold input; I2 output; I3 output
function [I1, I2, I3] = EMS_Controller(SOC1, SOC2, SOC3, Price, P_threshold)

Imax = 30;

SOC = [SOC1, SOC2, SOC3];
I = zeros(1,3);

% Check conditions
idx_low = find(SOC < 20);          % EVs below 20%
all_above_20 = all(SOC >= 20);

% -------------------------------
% MODE 1: HIGH PRICE + ANY SOC < 20
% -------------------------------
if Price > P_threshold && ~isempty(idx_low)
    
    % Find weakest EV
    [~, idx_min] = min(SOC);
    
    for i = 1:3
        if i == idx_min
            I(i) = Imax;          % charge weakest EV
        else
            I(i) = -Imax/2;       % others discharge
        end
    end

% -------------------------------
% MODE 2: LOW PRICE (GRID CHARGING)
% -------------------------------
elseif Price < P_threshold
    
    for i = 1:3
        I(i) = Imax * (1 - SOC(i)/100);   % proportional charging
    end

% -------------------------------
% MODE 3: HIGH PRICE + ALL SOC > 20 (SELL TO GRID)
% -------------------------------
elseif Price > P_threshold && all_above_20
    
    for i = 1:3
        I(i) = -Imax;   % all discharge to grid
    end

else
    I = zeros(1,3);
end

% Output
I1 = I(1);
I2 = I(2);
I3 = I(3);

end
